simulink model "lab9"  (R2019a)
settings: Solver=VariableStepAuto  StartTime=0.0  StopTime=100  RelTol=1e-3
settings Model: Creator=sumli  LastModifiedBy=sumli

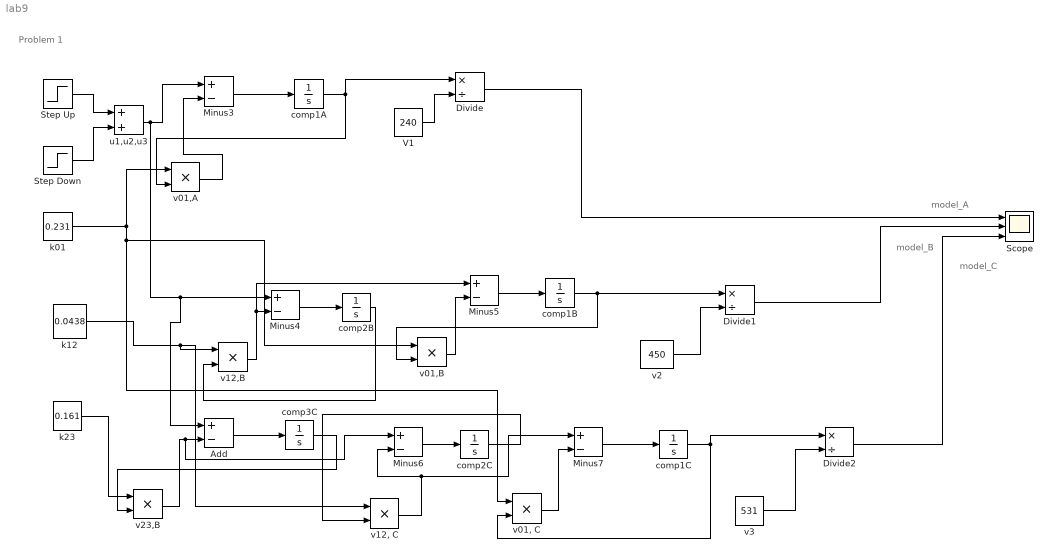
== system lab9 ==
  note: model_A
  note: Problem 1
  note: model_B
  note: model_C
  Add : Sum  Inputs=+-
  Divide : Product  Inputs=*/
  Divide1 : Product  Inputs=*/
  Divide2 : Product  Inputs=*/
  Minus{3..7} (5 alike) : Sum  Inputs=+-
  Scope : Scope  NumInputPorts=3
  Step Down : Step  Time=5.001  After=-300000000  SampleTime=0
  Step Up : Step  Time=5  After=300000000  SampleTime=0
  V1 : Constant  Value=240
  comp1A : Integrator
  comp1B : Integrator
  comp1C : Integrator
  comp2B : Integrator
  comp2C : Integrator
  comp3C : Integrator
  k01 : Constant  Value=0.231
  k12 : Constant  Value=0.0438
  k23 : Constant  Value=0.161
  u1,u2,u3 : Sum
  "v01, C" : Product
  v01,A : Product
  v01,B : Product
  "v12, C" : Product
  v12,B : Product
  v2 : Constant  Value=450
  v23,B : Product
  v3 : Constant  Value=531
  wires:
  Step Up/1 -> u1,u2,u3/1
  Step Down/1 -> u1,u2,u3/2
  Minus3/1 -> comp1A/1
  comp1A/1 -> v01,A/2, Divide/1
  u1,u2,u3/1 -> Minus3/1, Add/1, Minus4/1
  V1/1 -> Divide/2
  Divide/1 -> Scope/1
  Minus4/1 -> comp2B/1
  v01,A/1 -> Minus3/2
  k01/1 -> v01,B/1, "v01, C"/1, v01,A/1
  k12/1 -> "v12, C"/1, v12,B/1
  comp2B/1 -> v12,B/2
  v12,B/1 -> Minus5/1, Minus4/2
  Minus5/1 -> comp1B/1
  v01,B/1 -> Minus5/2
  comp1B/1 -> Divide1/1, v01,B/2
  v2/1 -> Divide1/2
  Divide1/1 -> Scope/2
  v23,B/1 -> Minus6/1, Add/2
  k23/1 -> v23,B/1
  Add/1 -> comp3C/1
  comp3C/1 -> v23,B/2
  Minus6/1 -> comp2C/1
  comp2C/1 -> "v12, C"/2
  "v12, C"/1 -> Minus7/1, Minus6/2
  Minus7/1 -> comp1C/1
  "v01, C"/1 -> Minus7/2
  comp1C/1 -> Divide2/1, "v01, C"/2
  v3/1 -> Divide2/2
  Divide2/1 -> Scope/3
